simulink model "wind_turbine"  (R2015a)
settings: Solver=ode45  StartTime=0.0  StopTime=50  RelTol=1e-3
libraries: simulink x1
settings Model: Creator=Administrador  LastModifiedBy=Administrador

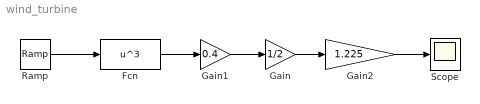
== system wind_turbine ==
  Fcn : Fcn  Expr=u^3
  Gain : Gain  Gain=1/2
  Gain1 : Gain  Gain=0.4
  Gain2 : Gain  Gain=1.225
  Ramp : simulink/Sources/Ramp  slope=1  start=5  X0=11
  Scope : Scope
  wires:
  Gain/1 -> Gain2/1
  Gain1/1 -> Gain/1
  Fcn/1 -> Gain1/1
  Gain2/1 -> Scope/1
  Ramp/1 -> Fcn/1
